simulink model "Problem__5"  (R2020b)
settings: Solver=VariableStepAuto  StartTime=0.0  StopTime=10.0  RelTol=1e-3
model workspace (MAT data in the model file):
  C = 1e-05
  R = 10
settings Model: Creator=Arvind Hishikar  LastModifiedBy=Arvind Hishikar

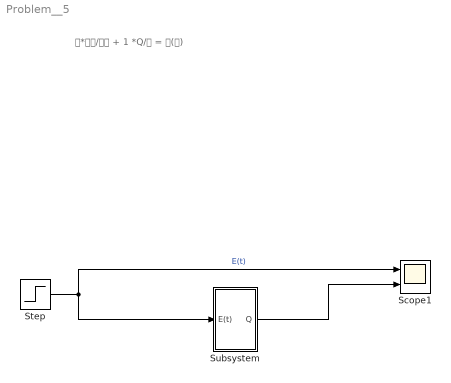
== system Problem__5 ==
  note: 𝑅*𝑑𝑄/𝑑𝑡 + 1 *Q/𝐶 = 𝐸(𝑡)
  Scope1 : Scope  NumInputPorts=2
  Step : Step  Time=0.1  After=5  SampleTime=0
  Subsystem : Subsystem
  wires:
  Step/1 -> Subsystem/1(E(t)), Scope1/1  "E(t)"
  Subsystem/1(Q) -> Scope1/2

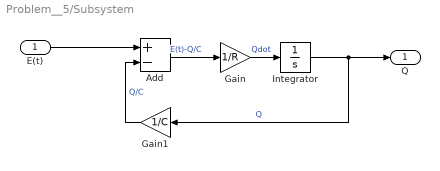
== system Problem__5/Subsystem ==
  E(t) : Inport
  Add : Sum  Inputs=+-
  Gain : Gain  Gain=1/R
  Gain1 : Gain  Gain=1/C
  Integrator : Integrator  InitialCondition=2  UpperSaturationLimit=5  LowerSaturationLimit=-5
  Q : Outport
  wires:
  Integrator/1 -> Q/1, Gain1/1  "Q"
  Add/1 -> Gain/1  "E(t)-Q/C"
  Gain1/1 -> Add/2  "Q/C"
  Gain/1 -> Integrator/1  "Qdot"
  E(t)/1 -> Add/1
